simulink library "ctrlAllocMatrix3CompCoef_cl"  (R2022a)
settings: Solver=VariableStepAuto  StartTime=0.0  StopTime=10.0  RelTol=1e-3
undefined symbols (not defined in the file or in its folder): fluidDensity, vhcl
libraries: hydroInversionCoef_cl x4, eulAng2RotMat_ul x1
settings Model: Creator=mcobb  LastModifiedBy=adabney
settings SolverCC: AlgebraicLoopSolver=TrustRegion
settings DataIOCC: ReturnWorkspaceOutputs=off
settings DebuggingCC: UnconnectedInputMsg=warning  UnconnectedOutputMsg=warning  UnconnectedLineMsg=warning  SFMachineParentedDataDiag=warning  ArithmeticOperatorsInVariantConditions=warning
settings SFSimCC: CustomCodeUndefinedFunction=UseInterfaceOnly

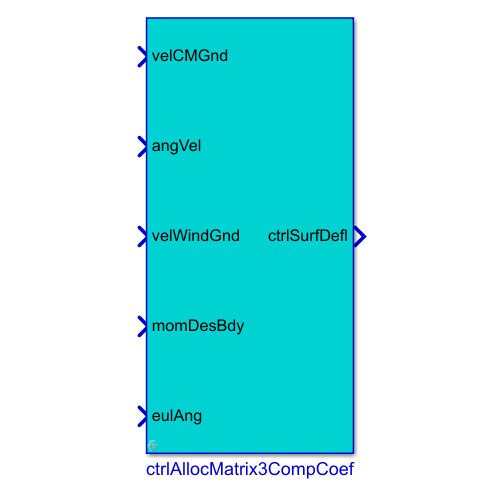
[thumbnail: Simulink's stored preview of the top-level diagram]
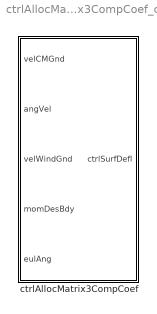
== system ctrlAllocMatrix3CompCoef_cl ==
  ctrlAllocMatrix3CompCoef : Subsystem  mask{aeroStruct=vhcl.struct('OCT.aeroSurf'), fluidDensity=fluidDensity, arms=vhcl.struct('OCT.thrAttch')}
      mask prompts: aeroStruct "Aerodynamic surface structure"; fluidDensity "Fluid density"; arms "Tether Attachment"
      settings: MinAlgLoopOccurrences=on
      mask TypeOptions aeroStruct: momentComponentVector/aeroStruct
      mask TypeOptions fluidDensity: momentComponentVector/fluidDensity

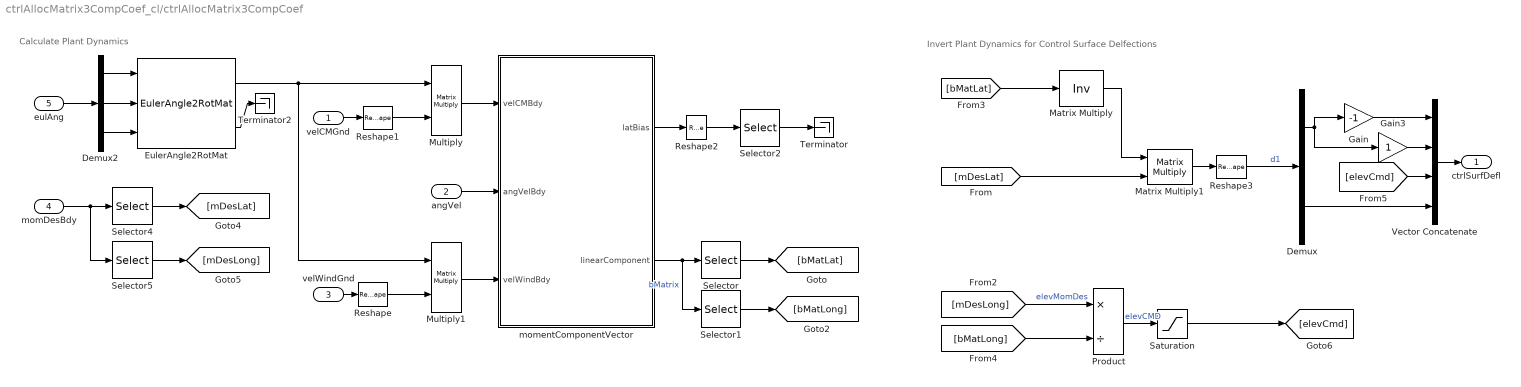
== system ctrlAllocMatrix3CompCoef_cl/ctrlAllocMatrix3CompCoef ==
  note: Invert Plant Dynamics for Control Surface Delfections
  note: Calculate Plant Dynamics
  velCMGnd : Inport
  angVel : Inport  Port=2
  velWindGnd : Inport  Port=3
  momDesBdy : Inport  Port=4
  eulAng : Inport  Port=5
  Demux : Demux  Outputs=2
  Demux2 : Demux  Outputs=3
  EulerAngle2RotMat : eulAng2RotMat_ul/EulerAngle2RotMat  SystemSampleTime=-1  VariantActivationTime=update diagram  Latency=0  AutoFrameSizeCalculation=off
  Gain : Gain  Gain=-1
  Gain3 : Gain
  Matrix Multiply : Product  Inputs=/  Multiplication=Matrix(*)
  Matrix Multiply1 : Product  Multiplication=Matrix(*)
  Multiply : Product  Multiplication=Matrix(*)
  Multiply1 : Product  Multiplication=Matrix(*)
  Product : Product  Inputs=*/
  Reshape : Reshape  OutputDimensionality=Column vector (2-D)
  Reshape1 : Reshape  OutputDimensionality=Column vector (2-D)
  Reshape2 : Reshape  OutputDimensionality=Column vector (2-D)
  Reshape3 : Reshape
  Saturation : Saturate  UpperLimit=30  LowerLimit=-30
  Selector : Selector  NumberOfDimensions=2  InputPortWidth=3  IndexOptions=Index vector (dialog),Index vector (dialog)  Indices=[1 3],[1 3]  OutputSizes=1,1
  Selector1 : Selector  NumberOfDimensions=2  InputPortWidth=3  IndexOptions=Index vector (dialog),Index vector (dialog)  Indices=2,2  OutputSizes=1,1
  Selector2 : Selector  InputPortWidth=3  IndexOptions=Index vector (dialog)  Indices=[1 3]  OutputSizes=1
  Selector4 : Selector  InputPortWidth=3  IndexOptions=Index vector (dialog)  Indices=[1 3]  OutputSizes=1
  Selector5 : Selector  InputPortWidth=3  IndexOptions=Index vector (dialog)  Indices=2  OutputSizes=1
  Terminator : Terminator
  Terminator2 : Terminator
  Vector Concatenate : Concatenate  NumInputs=4
  momentComponentVector : Subsystem  mask{aeroStruct=aeroStruct, fluidDensity=fluidDensity}
      mask prompts: aeroStruct "Aerodynamic surface structure"; fluidDensity "Fluid density"
      mask help:
      | Input must be an 1×N struct array with fields:
      |     refArea
      |     aeroCentPosVec
      |     spanUnitVec
      |     chordUnitVec
      |     CL
      |     CD
      |     alpha
      |     GainCL
      |     GainCD
      |
      | where N is the number of aerodynamic surfaces
  ctrlSurfDefl : Outport  VectorParamsAs1DForOutWhenUnconnected=off
  wires:
  Demux2/2 -> EulerAngle2RotMat/2
  eulAng/1 -> Demux2/1
  velWindGnd/1 -> Reshape/1
  EulerAngle2RotMat/2 -> Terminator2/1
  velCMGnd/1 -> Reshape1/1
  Multiply/1 -> momentComponentVector/1(velCMBdy)
  Reshape/1 -> Multiply1/2
  Demux2/1 -> EulerAngle2RotMat/1
  Reshape1/1 -> Multiply/2
  Demux2/3 -> EulerAngle2RotMat/3
  Multiply1/1 -> momentComponentVector/3(velWindBdy)
  EulerAngle2RotMat/1 -> Multiply1/1, Multiply/1
  Gain3/1 -> Vector Concatenate/2
  Vector Concatenate/1 -> ctrlSurfDefl/1
  Demux/1 -> Gain3/1, Gain/1
  Gain/1 -> Vector Concatenate/1
  Reshape3/1 -> Demux/1  "d1"
  angVel/1 -> momentComponentVector/2(angVelBdy)
  [mDesLat] -> Matrix Multiply1/2
  [bMatLat] -> Matrix Multiply/1
  Matrix Multiply1/1 -> Reshape3/1
  momentComponentVector/1(latBias) -> Reshape2/1
  momentComponentVector/2(linearComponent) -> Selector1/1, Selector/1  "bMatrix"
  Matrix Multiply/1 -> Matrix Multiply1/1
  Selector/1 -> [bMatLat]
  Selector1/1 -> [bMatLong]
  Selector2/1 -> Terminator/1
  Reshape2/1 -> Selector2/1
  Selector5/1 -> [mDesLong]
  Selector4/1 -> [mDesLat]
  momDesBdy/1 -> Selector5/1, Selector4/1
  [mDesLong] -> Product/1  "elevMomDes"
  [bMatLong] -> Product/2
  [elevCmd] -> Vector Concatenate/3
  Demux/2 -> Vector Concatenate/4
  Product/1 -> Saturation/1  "elevCMD"
  Saturation/1 -> [elevCmd]

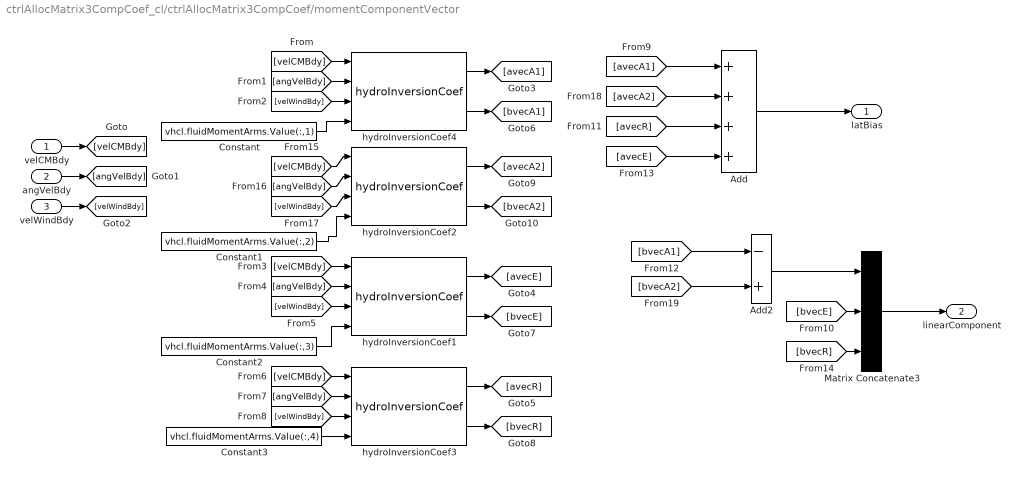
== system ctrlAllocMatrix3CompCoef_cl/ctrlAllocMatrix3CompCoef/momentComponentVector ==
  velCMBdy : Inport
  angVelBdy : Inport  Port=2
  velWindBdy : Inport  Port=3
  Add : Sum  Inputs=++++
  Add2 : Sum  Inputs=-+
  Constant : Constant  Value=vhcl.fluidMomentArms.Value(:,1)
  Constant1 : Constant  Value=vhcl.fluidMomentArms.Value(:,2)
  Constant2 : Constant  Value=vhcl.fluidMomentArms.Value(:,3)
  Constant3 : Constant  Value=vhcl.fluidMomentArms.Value(:,4)
  Matrix Concatenate3 : Concatenate  NumInputs=3  Mode=Multidimensional array  ConcatenateDimension=2
  hydroInversionCoef1 : hydroInversionCoef_cl/hydroInversionCoef  aeroStruct=vhcl.hStab
  hydroInversionCoef2 : hydroInversionCoef_cl/hydroInversionCoef  aeroStruct=vhcl.stbdWing
  hydroInversionCoef3 : hydroInversionCoef_cl/hydroInversionCoef  aeroStruct=vhcl.vStab
  hydroInversionCoef4 : hydroInversionCoef_cl/hydroInversionCoef  aeroStruct=vhcl.portWing
  latBias : Outport
  linearComponent : Outport  Port=2
  wires:
  velCMBdy/1 -> [velCMBdy]
  angVelBdy/1 -> [angVelBdy]
  velWindBdy/1 -> [velWindBdy]
  [velCMBdy] -> hydroInversionCoef4/1
  [angVelBdy] -> hydroInversionCoef4/2
  [velWindBdy] -> hydroInversionCoef4/3
  [angVelBdy] -> hydroInversionCoef3/2
  [velCMBdy] -> hydroInversionCoef3/1
  [velWindBdy] -> hydroInversionCoef3/3
  hydroInversionCoef4/1 -> [avecA1]
  hydroInversionCoef3/1 -> [avecR]
  hydroInversionCoef4/2 -> [bvecA1]
  hydroInversionCoef3/2 -> [bvecR]
  [avecR] -> Add/3
  [velWindBdy] -> hydroInversionCoef2/3
  hydroInversionCoef2/1 -> [avecA2]
  [angVelBdy] -> hydroInversionCoef2/2
  [velCMBdy] -> hydroInversionCoef2/1
  hydroInversionCoef2/2 -> [bvecA2]
  [avecA1] -> Add/1
  [avecA2] -> Add/2
  [bvecA1] -> Add2/1
  [bvecA2] -> Add2/2
  Constant/1 -> hydroInversionCoef4/4
  Constant1/1 -> hydroInversionCoef2/4
  Constant3/1 -> hydroInversionCoef3/4
  [bvecR] -> Matrix Concatenate3/3
  Matrix Concatenate3/1 -> linearComponent/1
  Add/1 -> latBias/1
  Add2/1 -> Matrix Concatenate3/1
  [bvecE] -> Matrix Concatenate3/2
  Constant2/1 -> hydroInversionCoef1/4
  hydroInversionCoef1/1 -> [avecE]
  [velCMBdy] -> hydroInversionCoef1/1
  [angVelBdy] -> hydroInversionCoef1/2
  hydroInversionCoef1/2 -> [bvecE]
  [avecE] -> Add/4
  [velWindBdy] -> hydroInversionCoef1/3
